simulink model "try_to_count"  (R2020a)
settings: Solver=FixedStepDiscrete  StartTime=0.0  StopTime=10  FixedStep=1e-3  RelTol=1e-3
libraries: simulink x1, dspswit3 x1
settings Model: Creator=Administrator  LastModifiedBy=Administrator

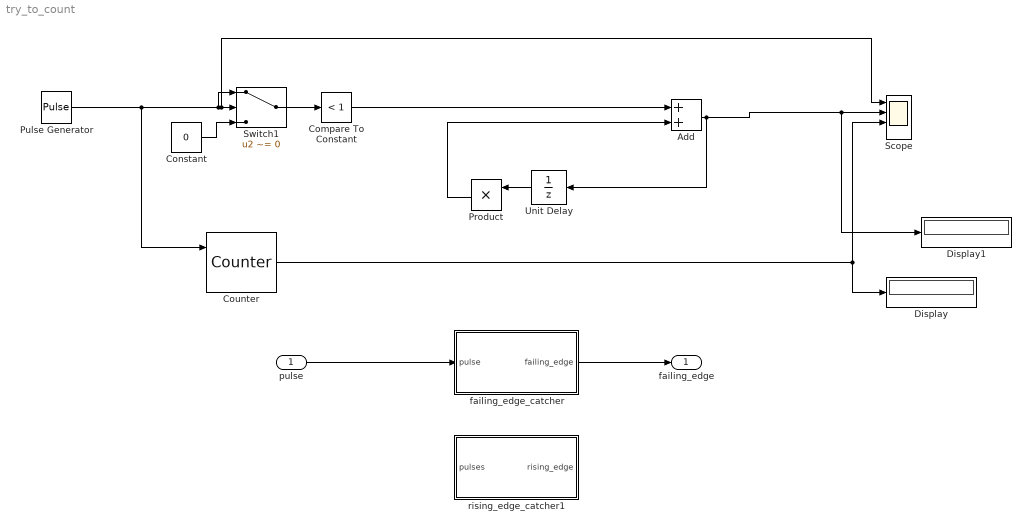
== system try_to_count ==
  pulse : Inport
  Add : Sum
  Compare To Constant : simulink/Logic and Bit Operations/Compare To Constant  relop=<  const=1  OutDataTypeStr=uint8
  Constant : Constant  Value=0
  Counter : dspswit3/Counter  Direction=Up  CountEvent=Falling edge  CounterSize=User defined  MaxCount=255  InitialCount=0  Output=Count  HitValue=32  ResetInput=on  SamplesPerFrame=1  Ts=1  CntDtype=double  HitDtype=Logical
  Display : Display
  Display1 : Display
  Product : Product  OutDataTypeStr=uint8
  Pulse Generator : DiscretePulseGenerator  PulseType=Time based  Period=1  PulseWidth=50
  Scope : Scope  NumInputPorts=4
  Switch1 : Switch  Criteria=u2 ~= 0
  Unit Delay : UnitDelay  SampleTime=.5  HasFrameUpgradeWarning=on
  failing_edge_catcher : Subsystem
  rising_edge_catcher1 : Subsystem
  failing_edge : Outport
  wires:
  Pulse Generator/1 -> Counter/1, Scope/1, Switch1/2, Switch1/1
  Counter/1 -> Display/1, Scope/3
  Compare To Constant/1 -> Add/1
  Switch1/1 -> Compare To Constant/1
  Constant/1 -> Switch1/3
  Add/1 -> Display1/1, Scope/2, Unit Delay/1
  Unit Delay/1 -> Product/1
  Product/1 -> Add/2
  pulse/1 -> failing_edge_catcher/1(pulse)
  failing_edge_catcher/1(failing_edge) -> failing_edge/1

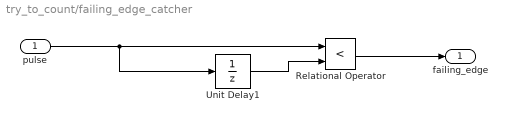
== system try_to_count/failing_edge_catcher ==
  pulse : Inport
  Relational Operator : RelationalOperator  Operator=<  OutDataTypeStr=boolean  RndMeth=Simplest
  Unit Delay1 : UnitDelay  SampleTime=-1  HasFrameUpgradeWarning=on
  failing_edge : Outport
  wires:
  pulse/1 -> Unit Delay1/1, Relational Operator/1
  Relational Operator/1 -> failing_edge/1
  Unit Delay1/1 -> Relational Operator/2

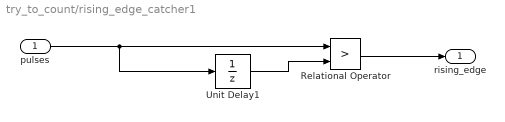
== system try_to_count/rising_edge_catcher1 ==
  pulses : Inport
  Relational Operator : RelationalOperator  Operator=>  OutDataTypeStr=boolean  RndMeth=Simplest
  Unit Delay1 : UnitDelay  SampleTime=-1  HasFrameUpgradeWarning=on
  rising_edge : Outport
  wires:
  Unit Delay1/1 -> Relational Operator/2
  Relational Operator/1 -> rising_edge/1
  pulses/1 -> Relational Operator/1, Unit Delay1/1
